simulink model "whitenoise_sim"  (Simulink 6.6)
settings: Solver=ode45  StartTime=0.0  StopTime=10.0  RelTol=1e-3
settings Model: Creator=mgilson  LastModifiedBy=mgilson  ExtModeAutoUpdateStatusClock=off

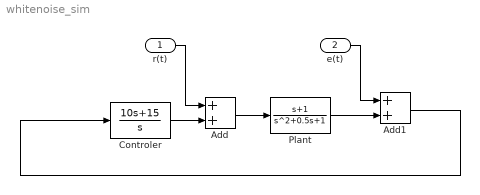
== system whitenoise_sim ==
  r(t) : Inport
  e(t) : Inport  Port=2
  Add : Sum  OutScaling=2^-10
  Add1 : Sum  OutScaling=2^-10
  Controler : TransferFcn  Numerator=[10 15]  Denominator=[1 0]
  Plant : TransferFcn  Numerator=[1 1]  Denominator="[1  0.5 1]"
  wires:
  Controler/1 -> Add/2
  Add/1 -> Plant/1
  Plant/1 -> Add1/2
  Add1/1 -> Controler/1
  r(t)/1 -> Add/1
  e(t)/1 -> Add1/1
